simulink model "SIM_CSTR_NOMINAL"  (R2023b)
settings: Solver=VariableStepAuto  StartTime=0.0  StopTime=30  RelTol=1e-3
values from neighbouring files (symbols this model uses):
  Ts = 0.05    [NMPC_CSTR.m]
  u0 = 300    [NMPC_CSTR.m]
libraries: mpclib x1, SignalEditorBlockLib x1
settings Model: Creator=DELL  LastModifiedBy=akeebismail

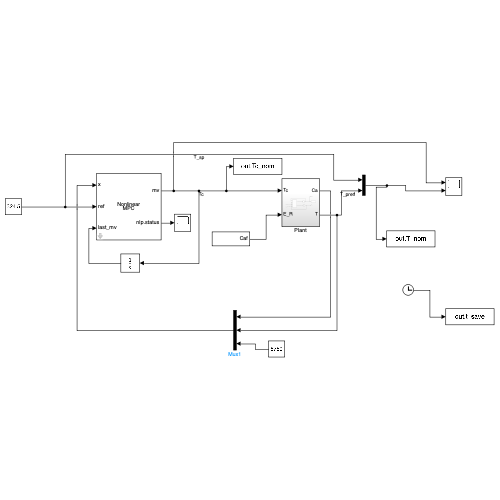
[thumbnail: Simulink's stored preview of the top-level diagram]
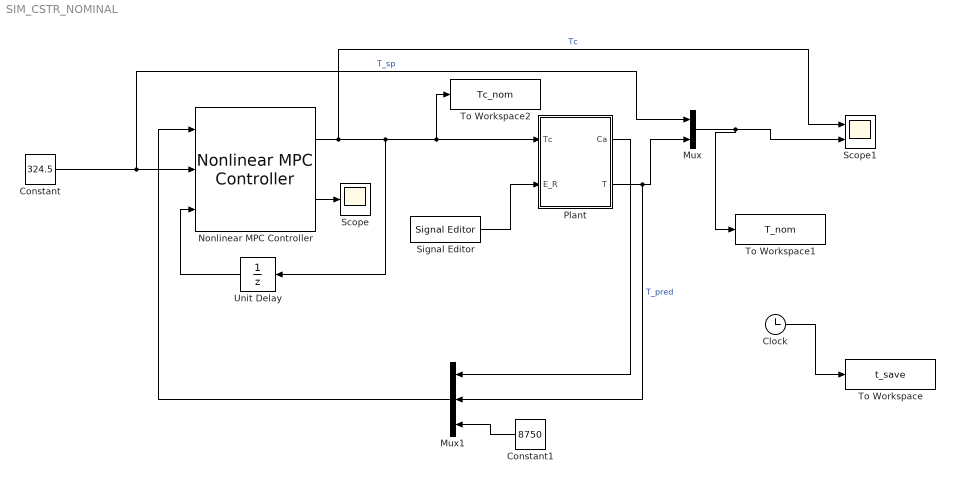
== system SIM_CSTR_NOMINAL ==
  Clock : Clock
  Constant : Constant  Value=324.5
  Constant1 : Constant  Value=8750
  Mux : Mux  Inputs=2
  Mux1 : Mux  Inputs=3
  Nonlinear MPC Controller : mpclib/Nonlinear MPC Controller  nlmpcobj=nlobj  UseObjectTs=on  UseMEX=off  md_enabled=off  mvtarget_enabled=off  param_enabled=off  cost_enabled=off  mvseq_enabled=off  stateseq_enabled=off  ovseq_enabled=off  slack_enabled=off  status_enabled=on  ov_min=off  ov_max=off  mv_min=off  mv_max=off  mvrate_min=off  mvrate_max=off  state_min=off  state_max=off  ov_weight=off  mv_weight=off  mvrate_weight=off  ecr_weight=off  nlp_initialize=off
  Plant : Subsystem
  Scope : Scope
  Scope1 : Scope  NumInputPorts=2
  Signal Editor : SignalEditorBlockLib/Signal Editor  FileName=Caf.mat  ActiveScenario=Scenario  ActiveSignal=Caf  IsBus=off  OutputBusObjectStr=Bus: BusObject  SampleTime=Ts  Interpolate=off  ZeroCross=off  OutputAfterFinalValue=Setting to zero  Unit=inherit  PreserveSignalName=on  ApplySigPropsToAllScenarios=on  ApplySigPropsToAllSignals=off
  To Workspace : ToWorkspace  VariableName=t_save  SaveFormat=Timeseries  SampleTime=Ts
  To Workspace1 : ToWorkspace  VariableName=T_nom  SaveFormat=Timeseries  SampleTime=Ts
  To Workspace2 : ToWorkspace  VariableName=Tc_nom  SaveFormat=Timeseries  SampleTime=Ts
  Unit Delay : UnitDelay  InitialCondition=u0  SampleTime=Ts  HasFrameUpgradeWarning=on
  wires:
  Constant/1 -> Mux/1, Nonlinear MPC Controller/2  "T_sp"
  Mux1/1 -> Nonlinear MPC Controller/1
  Nonlinear MPC Controller/1 -> To Workspace2/1, Plant/1(Tc), Unit Delay/1, Scope1/1  "Tc"
  Plant/2(T) -> Mux1/2, Mux/2  "T_pred"
  Nonlinear MPC Controller/2 -> Scope/1
  Mux/1 -> To Workspace1/1, Scope1/2
  Unit Delay/1 -> Nonlinear MPC Controller/3
  Signal Editor/1 -> Plant/2(E_R)
  Plant/1(Ca) -> Mux1/1
  Constant1/1 -> Mux1/3
  Clock/1 -> To Workspace/1

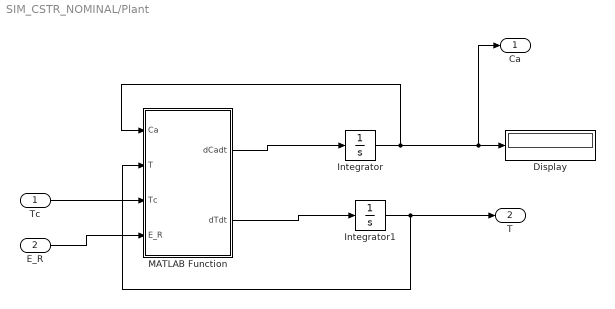
== system SIM_CSTR_NOMINAL/Plant ==
  Tc : Inport
  E_R : Inport  Port=2
  Display : Display
  Integrator : Integrator
  Integrator1 : Integrator  InitialCondition=300
  MATLAB Function : MATLAB Function  TreatAsAtomicUnit=on
  Ca : Outport
  T : Outport  Port=2
  wires:
  Integrator1/1 -> T/1, MATLAB Function/2(T)
  MATLAB Function/2(dTdt) -> Integrator1/1
  Integrator/1 -> Ca/1, Display/1, MATLAB Function/1(Ca)
  MATLAB Function/1(dCadt) -> Integrator/1
  Tc/1 -> MATLAB Function/3(Tc)
  E_R/1 -> MATLAB Function/4(E_R)

== matlab function SIM_CSTR_NOMINAL/Plant/MATLAB Function ==
  data: Ca input; dCadt output; T input; Tc input; dTdt output; E_R input
function [dCadt,dTdt] = fcn(Ca,T,Tc,E_R)

values = {100,5e4,350,100,1000,0.239,7.2e10,5e4,1};
[F,delta_H,Tf,V,rho,Cp,k0,U_A,Caf] = values{:};

% Rate constant (Arrhenius equation)
        k = k0 * exp(-E_R / T);
        
        % Mass balance for Ca
        dCadt = F/V * (Caf - Ca) - k * Ca;
        
        % Energy balance for T
        dTdt = F/V * (Tf - T) + (delta_H / (rho * Cp)) * k * Ca + (U_A / (rho * Cp * V)) * (Tc - T);


end
